simulink model "roll_control_pid"  (R2025b)
settings: Solver=VariableStepAuto  StartTime=0.0  StopTime=10.0  RelTol=1e-3
settings Model: Creator=srivatsan  LastModifiedBy=srivatsan

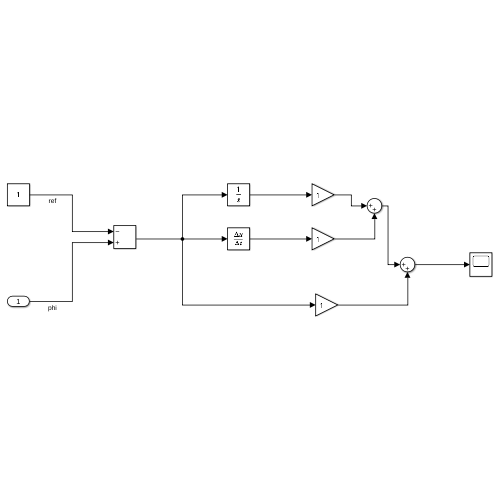
[thumbnail: Simulink's stored preview of the top-level diagram]
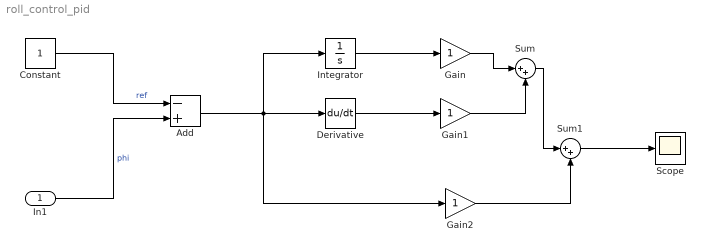
== system roll_control_pid ==
  In1 : Inport
  Add : Sum  Inputs=-+
  Constant : Constant
  Derivative : Derivative
  Gain : Gain
  Gain1 : Gain
  Gain2 : Gain
  Integrator : Integrator
  Scope : Scope
      settings: ActiveDisplayYMinimum=-22.190795480635238  ActiveDisplayYMaximum=2.55834951235724
  Sum : Sum  Inputs=|++
  Sum1 : Sum  Inputs=|++
  wires:
  In1/1 -> Add/2  "phi"
  Constant/1 -> Add/1  "ref"
  Add/1 -> Gain2/1, Derivative/1, Integrator/1
  Derivative/1 -> Gain1/1
  Integrator/1 -> Gain/1
  Gain/1 -> Sum/1
  Gain1/1 -> Sum/2
  Sum/1 -> Sum1/1
  Gain2/1 -> Sum1/2
  Sum1/1 -> Scope/1
